simulink model "DualMinSegBalance_Code_V31_DeadbandComp_PID"  (R2014a)
settings: Solver=FixedStepDiscrete  SolverMode=SingleTasking  StartTime=0.0  StopTime=inf  FixedStep=TS  RelTol=1e-3
values from neighbouring files (symbols this model uses):
  ES = -C2DEG*D2R    (= -0.00872664625997)    [NXT_ParametersDual.m]
  GS = GyroS*D2R    (= 0.000532632218016)    [NXT_ParametersDual.m]
  Rw = .02    (= 0.02)    [NXT_ParametersDual.m]
  TS = 0.01    [NXT_ParametersDual.m]
undefined symbols (not defined in the file or in its folder): DiscIntNeverNeededParam
libraries: arduinolib x3, simulink x1
settings Model: FPTRunName=FPA_Reference  ExtModeTrigDuration=2  Creator=Alec  LastModifiedBy=Brian
settings OptimizationCC: ExpressionDepthLimit=2147483647  OptimizeModelRefInitCode=on  LifeSpan=1
settings DebuggingCC: UnderspecifiedInitializationDetection=Classic  SolverPrmCheckMsg=none  StateNameClashWarn=warning
settings HardwareCC: ProdBitPerInt=16  ProdBitPerPointer=8  ProdIntDivRoundTo=Zero  ProdEndianess=LittleEndian  ProdWordSize=8  ProdHWDeviceType=Atmel->AVR
settings RTWCC: SystemTargetFile=realtime.tlc  GenerateMakefile=off  TemplateMakefile=realtime.tmf  Description=Real-Time Toolbox  RTWVerbose=off  ProcessScript=realtime_make_rtw_hook
settings CodeAppCC: CustomSymbolStrType=$N$R$M  InternalIdentifier=Classic
settings STFCustomTargetCC: TargetLibSuffix=.a  GenerateSampleERTMain=on  ConcurrentExecutionCompliant=off  GeneratePreprocessorConditionals=Use local settings  ERTCustomFileBanners=on  SupportNonInlinedSFcns=off  SupportVariableSizeSignals=on  MATLABClassNameForMDSCustomization=Simulink.SoftwareTarget.ERTCustomization  GRTInterface=off  SystemTargetFile=realtime.tlc
settings ERTTargetCC: CombineOutputUpdateFcns=off  SupportContinuousTime=on  SupportVariableSizeSignals=on  ExtModeTransport=3  ExtModeMexFile=ext_serial_win32_comm  ExtModeMexArgs=0 5 115200  ERTSrcFileBannerTemplate=realtime_code_template.cgt  ERTHdrFileBannerTemplate=realtime_code_template.cgt  ERTDataSrcFileTemplate=realtime_code_template.cgt  ERTDataHdrFileTemplate=realtime_code_template.cgt  ERTCustomFileTemplate=realtime_file_process.tlc

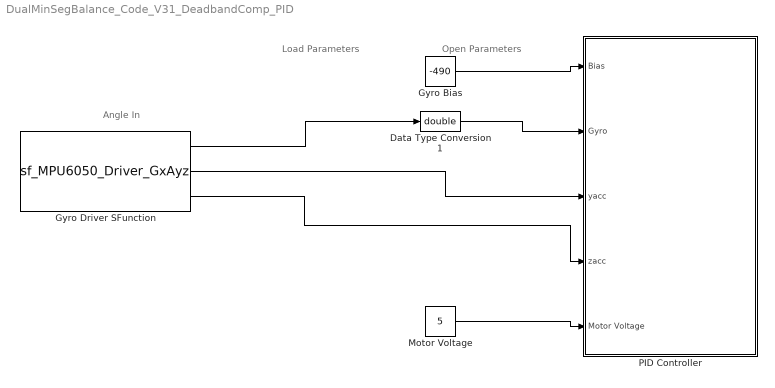
== system DualMinSegBalance_Code_V31_DeadbandComp_PID ==
  note: Load Parameters
  note: Open Parameters
  note: Angle In
  Data Type Conversion1 : DataTypeConversion  OutDataTypeStr=double
  Gyro Bias : Constant  Value=-490
  Gyro Driver SFunction : S-Function  InitFcn=try, set_param(gcb,'FunctionName','sf_MPU6050_Driver_GxAyz'), end  FunctionName=sf_MPU6050_Driver_GxAyz  SFunctionModules=sf_MPU6050_Driver_GxAyz_wrapper  EnableBusSupport=off  mask(S-Function Builder){}
      mask help: Simulink:masks:SFunctionBuilder_MD
      mask init:
      | val = [[.9  0.75 0.75 1 1 .9 .9 1]',[1 1 0.75 0.75 .9 .9 1 .9]'];try , sys = get_param(gcb,'SfunBuilderFcnName');if isempty(sys), sys = get_param(gcb,'FunctionName'); end,catch, sys = get_param(gcb,'FunctionName'); end
      settings: CopyFcn=set_param(gcbh,'LinkStatus','none')  PreSaveFcn=try, set_param(gcb,'FunctionName','sf_MPU6050_Driver_GxAyz'), end  OpenFcn=sfunctionwizard(gcbh)
      mask Display: plot(val(:,1),val(:,2)),disp(sys), port_label('output',1,'x_vel'), port_label('output',2,'y_acc'), port_label('output',3,'z_acc')
  Motor Voltage : Constant  Value=5
  PID Controller : Subsystem
  wires:
  Gyro Driver SFunction/1 -> Data Type Conversion1/1
  Data Type Conversion1/1 -> PID Controller/2(Gyro)
  Gyro Driver SFunction/2 -> PID Controller/3("yacc ")
  Gyro Driver SFunction/3 -> PID Controller/4("zacc ")
  Gyro Bias/1 -> PID Controller/1(Bias)
  Motor Voltage/1 -> PID Controller/5(Motor Voltage)

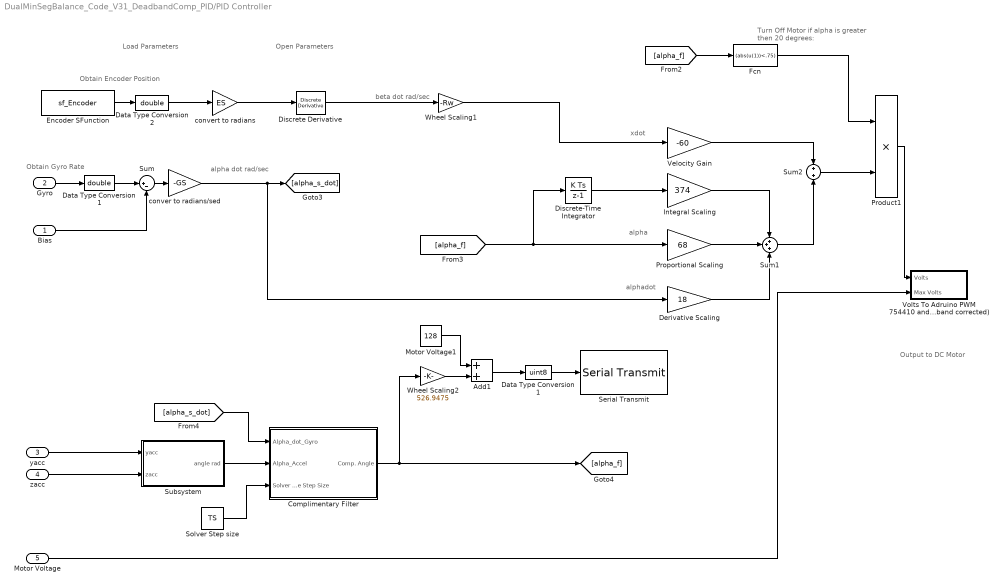
== system DualMinSegBalance_Code_V31_DeadbandComp_PID/PID Controller ==
  note: Turn Off Motor if alpha is
      | greater then 20 degrees:
  note: Output to DC Motor
  note: Obtain Gyro Rate
  note: alpha dot
      | rad/sec
  note: alpha
  note: alphadot
  note: Load Parameters
  note: Open Parameters
  note: Obtain Encoder Position
  note: xdot
  note: beta dot
      | rad/sec
  Bias : Inport
  Gyro : Inport  Port=2
  "yacc " : Inport  Port=3
  "zacc " : Inport  Port=4
  Motor Voltage : Inport  Port=5
  Add1 : Sum
  Complimentary Filter : Subsystem
  Data Type Conversion1 : DataTypeConversion  OutDataTypeStr=double
  Data Type Conversion2 : DataTypeConversion  OutDataTypeStr=double
  Data Type Conversion1 : DataTypeConversion  OutDataTypeStr=uint8  RndMeth=Nearest
  Derivative Scaling : Gain  Gain=18
  Discrete Derivative : simulink/Discrete/Discrete Derivative  gainval=1.0  ICPrevScaledInput=0.0  InputProcessing=Inherited  OutMin=[]  OutMax=[]  OutDataType=fixdt(1, 16)  OutScaling=2^-10  DoSatur=off
  Discrete-Time Integrator : DiscreteIntegrator  SampleTime=-1  LimitOutput=on  UpperSaturationLimit=3/374  LowerSaturationLimit=-3/374  ICPrevOutput=DiscIntNeverNeededParam  ICPrevScaledInput=DiscIntNeverNeededParam
  Encoder SFunction : S-Function  InitFcn=try, set_param(gcb,'FunctionName','sf_Encoder'), end  FunctionName=sf_Encoder  Parameters=uint8(0),uint8(18),uint8(19)  SFunctionModules=sf_Encoder_wrapper  EnableBusSupport=off  mask(S-Function Builder){}
      mask init: same as DualMinSegBalance_Code_V31_DeadbandComp_PID/Gyro Driver SFunction
      settings: CopyFcn=set_param(gcbh,'LinkStatus','none')  PreSaveFcn=try, set_param(gcb,'FunctionName','sf_Encoder'), end  OpenFcn=sfunctionwizard(gcbh)
      mask Display: plot(val(:,1),val(:,2)),disp(sys), port_label('output',1,'pos')
  Fcn : Fcn  Expr=(abs(u(1))<.75)
  Integral Scaling : Gain  Gain=374
  Motor Voltage1 : Constant  Value=128
  Product1 : Product  RndMeth=Zero
  Proportional Scaling : Gain  Gain=68
  Serial Transmit : arduinolib/Serial Transmit  portNumber=2
  Solver Step size : Constant  Value=TS
  Subsystem : Subsystem
  Sum : Sum  Inputs=|+-
  Sum1 : Sum  Inputs=+++
  Sum2 : Sum  Inputs=+|+
  Velocity Gain : Gain  Gain=-60
  Volts To Adruino PWM 754410 and Motor1 (Deadband corrected) : Subsystem
  Wheel Scaling1 : Gain  Gain=-Rw
  Wheel Scaling2 : Gain  Gain=526.9475
  conver to radians/sed : Gain  Gain=-GS
  convert to radians : Gain  Gain=ES  OutDataTypeStr=double
  wires:
  Bias/1 -> Sum/2
  Sum/1 -> conver to radians/sed/1
  Data Type Conversion1/1 -> Sum/1
  Gyro/1 -> Data Type Conversion1/1
  [alpha_f] -> Fcn/1
  "yacc "/1 -> Subsystem/1(yacc)
  "zacc "/1 -> Subsystem/2(zacc)
  Fcn/1 -> Product1/1
  Subsystem/1(angle rad) -> Complimentary Filter/2(Alpha_Accel)
  [alpha_s_dot] -> Complimentary Filter/1(Alpha_dot_Gyro)
  Solver Step size/1 -> Complimentary Filter/3(Solver Time Step Size)
  Complimentary Filter/1(Comp. Angle) -> Wheel Scaling2/1, [alpha_f]
  Product1/1 -> Volts To Adruino PWM 754410 and Motor1 (Deadband corrected)/1(Volts)
  Motor Voltage/1 -> Volts To Adruino PWM 754410 and Motor1 (Deadband corrected)/2(Max Volts)
  Data Type Conversion1/1 -> Serial Transmit/1
  Add1/1 -> Data Type Conversion1/1
  Wheel Scaling2/1 -> Add1/2
  Motor Voltage1/1 -> Add1/1
  conver to radians/sed/1 -> Derivative Scaling/1, [alpha_s_dot]
  [alpha_f] -> Discrete-Time Integrator/1, Proportional Scaling/1
  Proportional Scaling/1 -> Sum1/2
  Derivative Scaling/1 -> Sum1/3
  Encoder SFunction/1 -> Data Type Conversion2/1
  Data Type Conversion2/1 -> convert to radians/1
  Sum1/1 -> Sum2/2
  Sum2/1 -> Product1/2
  Wheel Scaling1/1 -> Velocity Gain/1
  Discrete-Time Integrator/1 -> Integral Scaling/1
  Integral Scaling/1 -> Sum1/1
  convert to radians/1 -> Discrete Derivative/1
  Discrete Derivative/1 -> Wheel Scaling1/1
  Velocity Gain/1 -> Sum2/1

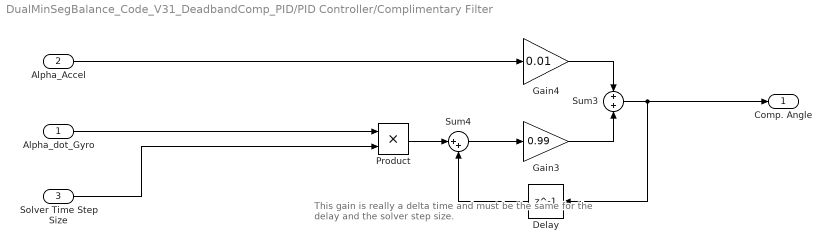
== system DualMinSegBalance_Code_V31_DeadbandComp_PID/PID Controller/Complimentary Filter ==
  note: This gain is really a delta time and must be the same for
      | the delay and the solver step size.
  Alpha_dot_Gyro : Inport
  Alpha_Accel : Inport  Port=2
  Solver Time Step Size : Inport  Port=3
  Delay : Delay  DelayLength=1  InitialCondition=0
  Gain3 : Gain  Gain=0.99
  Gain4 : Gain  Gain=0.01
  Product : Product
  Sum3 : Sum
  Sum4 : Sum  Inputs=|++
  Comp. Angle : Outport
  wires:
  Gain3/1 -> Sum3/2
  Gain4/1 -> Sum3/1
  Sum3/1 -> Comp. Angle/1, Delay/1
  Sum4/1 -> Gain3/1
  Delay/1 -> Sum4/2
  Product/1 -> Sum4/1
  Alpha_Accel/1 -> Gain4/1
  Alpha_dot_Gyro/1 -> Product/1
  Solver Time Step Size/1 -> Product/2

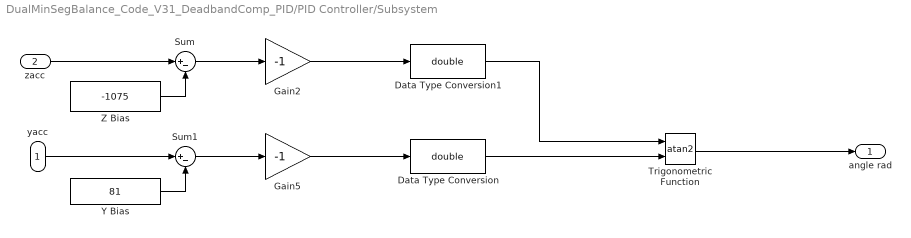
== system DualMinSegBalance_Code_V31_DeadbandComp_PID/PID Controller/Subsystem ==
  yacc : Inport
  zacc : Inport  Port=2
  Data Type Conversion : DataTypeConversion  OutDataTypeStr=double
  Data Type Conversion1 : DataTypeConversion  OutDataTypeStr=double
  Gain2 : Gain  Gain=-1
  Gain5 : Gain  Gain=-1
  Sum : Sum  Inputs=|+-
  Sum1 : Sum  Inputs=|+-
  Trigonometric Function : Trigonometry  Operator=atan2
  Y Bias : Constant  Value=81
  Z Bias : Constant  Value=-1075
  angle rad : Outport
  wires:
  Z Bias/1 -> Sum/2
  Y Bias/1 -> Sum1/2
  Trigonometric Function/1 -> angle rad/1
  Data Type Conversion1/1 -> Trigonometric Function/1
  Data Type Conversion/1 -> Trigonometric Function/2
  zacc/1 -> Sum/1
  yacc/1 -> Sum1/1
  Gain2/1 -> Data Type Conversion1/1
  Sum/1 -> Gain2/1
  Sum1/1 -> Gain5/1
  Gain5/1 -> Data Type Conversion/1

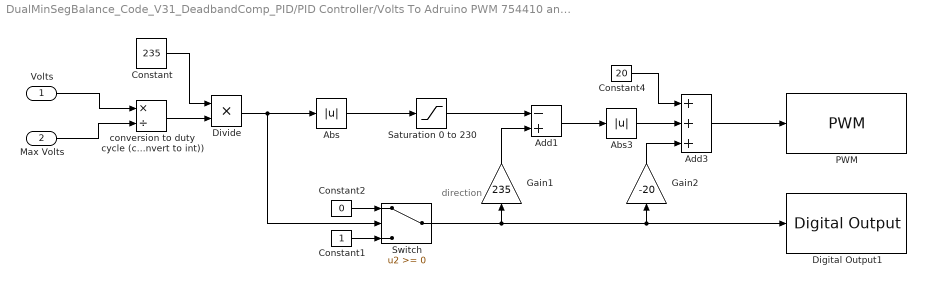
== system DualMinSegBalance_Code_V31_DeadbandComp_PID/PID Controller/Volts To Adruino PWM 754410 and Motor1 (Deadband corrected) ==
  note: direction
  Volts : Inport
  Max Volts : Inport  Port=2
  Abs : Abs
  Abs3 : Abs
  Add1 : Sum  Inputs=-+
  Add3 : Sum  Inputs=+++
  Constant : Constant  Value=235
  Constant1 : Constant
  Constant2 : Constant  Value=0
  Constant4 : Constant  Value=20
  Digital Output1 : arduinolib/Digital Output  pinNumber=8
  Divide : Product  Inputs=**
  Gain1 : Gain  Gain=235
  Gain2 : Gain  Gain=-20
  PWM : arduinolib/PWM  pinNumber=6
  Saturation 0 to 230 : Saturate  UpperLimit=230  LowerLimit=0
  Switch : Switch
  conversion to duty cycle (convert to int)) : Product  Inputs=*/  OutDataTypeStr=double
  wires:
  Abs/1 -> Saturation 0 to 230/1
  Saturation 0 to 230/1 -> Add1/1
  Add1/1 -> Abs3/1
  Gain1/1 -> Add1/2
  Constant1/1 -> Switch/3
  Constant2/1 -> Switch/1
  Switch/1 -> Gain1/1, Gain2/1, Digital Output1/1
  Abs3/1 -> Add3/2
  Add3/1 -> PWM/1
  Constant4/1 -> Add3/1
  Volts/1 -> conversion to duty cycle (convert to int))/1
  Max Volts/1 -> conversion to duty cycle (convert to int))/2
  Divide/1 -> Switch/2, Abs/1
  conversion to duty cycle (convert to int))/1 -> Divide/2
  Constant/1 -> Divide/1
  Gain2/1 -> Add3/3
